simulink model "ROBOT"  (R2015a)
settings: Solver=ode45  SolverMode=SingleTasking  StartTime=0.0  StopTime=Tfinal  RelTol=1e-3
values from neighbouring files (symbols this model uses):
  Tem = 0.001    [Circular.m]    (also in Lineal.m)
undefined symbols (not defined in the file or in its folder): mgd, mgi
libraries: simulink x1
settings Model: CovMetricSettings=dwe  CovHtmlReporting=off  covSaveCumulativeToWorkspaceVar=off  CovSaveSingleToWorkspaceVar=off  CovExternalEMLEnable=on  Creator=Shadow  LastModifiedBy=Shadow
settings DataIOCC: LimitDataPoints=off  SaveFormat=Dataset  ReturnWorkspaceOutputs=on
settings DebuggingCC: SFUnexpectedBacktrackingDiag=error  SFNoUnconditionalDefaultTransitionDiag=error
settings HardwareCC: ProdBitPerPointer=64  ProdLargestAtomicFloat=Float  ProdIntDivRoundTo=Zero  ProdEndianess=LittleEndian  ProdHWDeviceType=Specified
settings ModelReferenceCC: PropagateSignalLabelsOutOfModel=on
settings SFSimCC: SimUseLocalCustomCode=on
settings RTWCC: RTWUseLocalCustomCode=on
settings GRTTargetCC: TargetLangStandard=C99 (ISO)

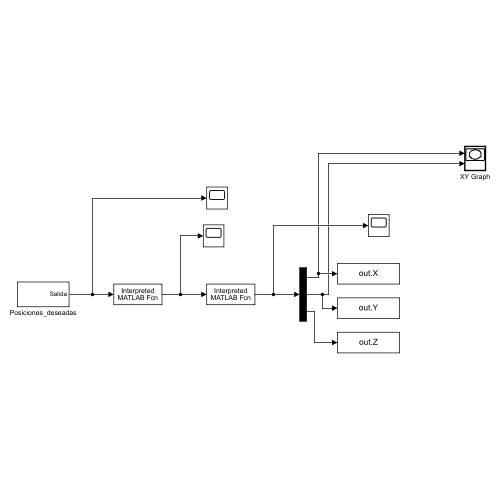
[thumbnail: Simulink's stored preview of the top-level diagram]
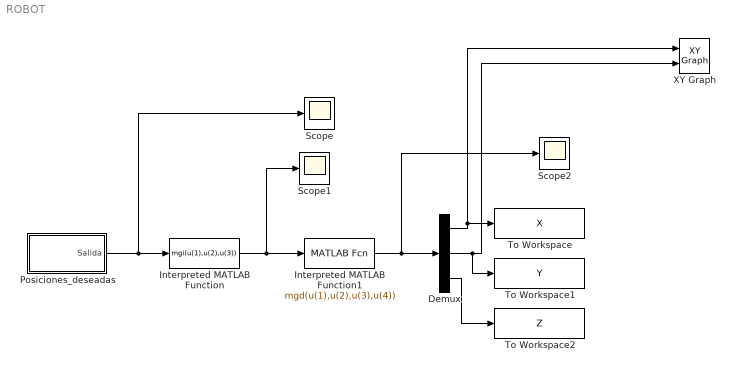
== system ROBOT ==
  Demux : Demux  Outputs=3
  Interpreted MATLAB Function : MATLABFcn  MATLABFcn=mgi(u(1),u(2),u(3))
  Interpreted MATLAB Function1 : MATLABFcn  MATLABFcn=mgd(u(1),u(2),u(3),u(4))
  Posiciones_deseadas : Subsystem
  Scope : Scope
      settings: TimeRange=auto  MaxDataPoints=5000  SaveToWorkspace=off  SaveName=ScopeData  YMin=0.275  YMax=0.525  SampleTime=-1
  Scope1 : Scope
      settings: TimeRange=auto  MaxDataPoints=5000  SaveToWorkspace=off  YMin=-1.20389  YMax=1.20389  SampleTime=-1
  Scope2 : Scope
      settings: TimeRange=auto  MaxDataPoints=5000  SaveToWorkspace=off  SaveName=ScopeData2  YMin=0.275  YMax=0.525  SampleTime=-1
  To Workspace : ToWorkspace  VariableName=X
  To Workspace1 : ToWorkspace  VariableName=Y
  To Workspace2 : ToWorkspace  VariableName=Z
  XY Graph : simulink/Sinks/XY Graph  xmin=-1  xmax=1  ymin=-1  ymax=1  st=-1
  wires:
  Interpreted MATLAB Function1/1 -> Scope2/1, Demux/1
  Interpreted MATLAB Function/1 -> Scope1/1, Interpreted MATLAB Function1/1
  Posiciones_deseadas/1(Salida) -> Scope/1, Interpreted MATLAB Function/1
  Demux/1 -> XY Graph/1, To Workspace/1
  Demux/2 -> XY Graph/2, To Workspace1/1
  Demux/3 -> To Workspace2/1

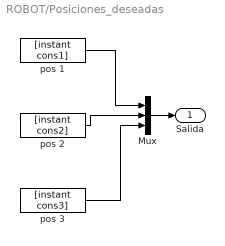
== system ROBOT/Posiciones_deseadas ==
  Mux : Mux  Inputs=3
  pos 1 : FromWorkspace  VariableName=[instant cons1]  SampleTime=Tem  ZeroCross=off
  pos 2 : FromWorkspace  VariableName=[instant cons2]  SampleTime=Tem  ZeroCross=off
  pos 3 : FromWorkspace  VariableName=[instant cons3]  SampleTime=Tem  ZeroCross=off
  Salida : Outport
  wires:
  pos 1/1 -> Mux/1
  pos 2/1 -> Mux/2
  pos 3/1 -> Mux/3
  Mux/1 -> Salida/1
